simulink model "evaporator"  (R2018b)
settings: Solver=VariableStepAuto  StartTime=0.0  StopTime=10.0  RelTol=1e-3
settings Model: Creator=smf52  LastModifiedBy=art58

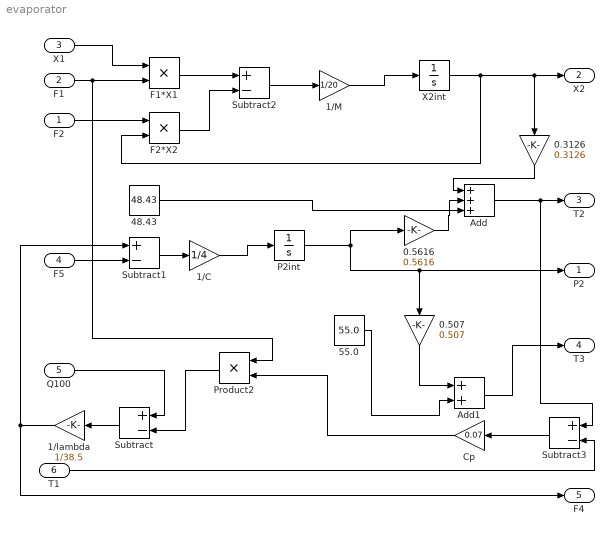
== system evaporator ==
  F2 : Inport
  F1 : Inport  Port=2
  "X1 " : Inport  Port=3
  F5 : Inport  Port=4
  Q100 : Inport  Port=5
  T1 : Inport  Port=6
  0.3126 : Gain  Gain=0.3126
  0.507 : Gain  Gain=0.507
  0.5616 : Gain  Gain=0.5616
  1/C : Gain  Gain=1/4
  1/M : Gain  Gain=1/20
  1/lambda : Gain  Gain=1/38.5
  48.43 : Constant  Value=48.43
  55.0 : Constant  Value=55.0
  Add : Sum  Inputs=+++
  Add1 : Sum
  Cp : Gain  Gain=0.07
  F1*X1 : Product
  F2*X2 : Product
  P2int : Integrator
  Product2 : Product
  Subtract{,1..3} (4 alike) : Sum  Inputs=+-
  X2int : Integrator
  "P2 " : Outport
  X2 : Outport  Port=2
  T2 : Outport  Port=3
  "T3 " : Outport  Port=4
  F4 : Outport  Port=5
  wires:
  F1/1 -> Product2/1, F1*X1/2
  "X1 "/1 -> F1*X1/1
  F2/1 -> F2*X2/1
  Subtract2/1 -> 1/M/1
  X2int/1 -> F2*X2/2, X2/1, 0.3126/1
  Subtract1/1 -> 1/C/1
  1/C/1 -> P2int/1
  P2int/1 -> 0.507/1, "P2 "/1, 0.5616/1
  Add/1 -> Subtract3/1, T2/1
  0.507/1 -> Add1/1
  Add1/1 -> "T3 "/1
  0.5616/1 -> Add/2
  0.3126/1 -> Add/1
  48.43/1 -> Add/3
  55.0/1 -> Add1/2
  T1/1 -> Subtract3/2
  Cp/1 -> Product2/2
  Product2/1 -> Subtract/2
  Q100/1 -> Subtract/1
  Subtract/1 -> 1/lambda/1
  F5/1 -> Subtract1/2
  1/lambda/1 -> F4/1, Subtract1/1
  F2*X2/1 -> Subtract2/2
  F1*X1/1 -> Subtract2/1
  Subtract3/1 -> Cp/1
  1/M/1 -> X2int/1
